simulink subsystem "Final_Project"  (R2024a)
settings: Solver=VariableStepAuto  StartTime=0.0  StopTime=10.0  RelTol=1e-3
undefined symbols (not defined in the file or in its folder): waypoints
libraries: CarMaker4SL x82
(part 3 of 4)

== matlab function Final_Project/Lib_Driving/Subsystem/MATLAB Function1 ==
  data: ego input Bus: EgoStateBus; front_dist output double; lanes input Bus: ParsedLaneBus; traffic input; target_speed input double; ego_lane_id input int32; front_v output double; left_clear output boolean; right_clear output boolean; ego_v input
function [front_dist, front_v, left_clear, right_clear] = traffic_detector(ego, lanes, traffic, target_speed, ego_lane_id, ego_v)
%#codegen
% traffic : Obstacle_Info_Bus
% 내부 구조 예:
%   traffic.t16.x, traffic.t16.y, traffic.t16.vx, traffic.t16.vy
%   ...
%   traffic.t28.x, traffic.t28.y, traffic.t28.vx, traffic.t28.vy
%
% 주의:
%   오류 고친 버전 기준으로 ego_v 입력을 추가함.
%   target_speed는 배선 호환용으로 남겨두지만, 거리 판단에는 ego_v를 사용함.

    unused_target_speed = target_speed; %#ok<NASGU>

    % ============================================================
    % 0. 출력 초기화
    % ============================================================
    front_dist  = 1e9;
    front_v     = 0.0;
    left_clear  = true;
    right_clear = true;
    ego_lane    = int32(ego_lane_id);

    % ============================================================
    % 1. Ego unpack
    % ============================================================
    ego_x = ego.Car_Fr1_tx;
    ego_y = ego.Car_Fr1_ty;

    % ============================================================
    % 2. Lane unpack - 5차선
    % ============================================================
    x1 = lanes.x1; y1 = lanes.y1;
    x2 = lanes.x2; y2 = lanes.y2;
    x3 = lanes.x3; y3 = lanes.y3;
    x4 = lanes.x4; y4 = lanes.y4;
    x5 = lanes.x5; y5 = lanes.y5;

    % detector와 lane5 기준을 맞추기 위한 보정
    L5_OFFSET = 1.0;
    x5 = x5 + L5_OFFSET;

    % ============================================================
    % 3. Ego 속도 기반 가변 탐색/안전거리
    % ============================================================
    v_ego_gap = abs(ego_v);

    % ego_v가 혹시 km/h로 들어오는 경우만 보호
    if v_ego_gap > 60.0
        v_ego_gap = v_ego_gap / 3.6;
    end

    % 같은 차선 앞차 탐색 거리
    LOOK_FRONT = calcLookFront(v_ego_gap);

    % 옆 차선 뒤쪽 안전거리
    CLEAR_BACK_MIN = 5.0;
    CLEAR_BACK_TG  = 0.5;
    CLEAR_BACK_MAX = 35.0;

    CLEAR_BACK = CLEAR_BACK_MIN + CLEAR_BACK_TG * v_ego_gap;

    if CLEAR_BACK > CLEAR_BACK_MAX
        CLEAR_BACK = CLEAR_BACK_MAX;
    end

    % 옆 차선 앞쪽 안전거리
    CLEAR_FRONT_MIN = 15.0;
    CLEAR_FRONT_TG  = 0.9;
    CLEAR_FRONT_MAX = 70.0;

    CLEAR_FRONT = CLEAR_FRONT_MIN + CLEAR_FRONT_TG * v_ego_gap;

    if CLEAR_FRONT > CLEAR_FRONT_MAX
        CLEAR_FRONT = CLEAR_FRONT_MAX;
    end

    % ============================================================
    % 4. Init
    % ============================================================
    front_dist = 1e9;
    front_v    = v_ego_gap;

    left_clear  = true;
    right_clear = true;

    % 도로 끝 차선에서는 없는 방향으로 차선변경 불가 처리
    if ego_lane >= int32(5)
        left_clear = false;
    end

    if ego_lane <= int32(1)
        right_clear = false;
    end

    % ============================================================
    % 5. Traffic_Info_16_Bus ~ Traffic_Info_28_Bus 직접 처리
    % ============================================================
    [front_dist, front_v, left_clear, right_clear] = check_one_signal( ...
        traffic.t16.x, traffic.t16.y, traffic.t16.vx, traffic.t16.vy, true, ...
        ego_x, ego_y, ego_lane, ...
        x1,y1,x2,y2,x3,y3,x4,y4,x5,y5, ...
        front_dist, front_v, left_clear, right_clear, ...
        LOOK_FRONT, CLEAR_BACK, CLEAR_FRONT);

    [front_dist, front_v, left_clear, right_clear] = check_one_signal( ...
        traffic.t17.x, traffic.t17.y, traffic.t17.vx, traffic.t17.vy, true, ...
        ego_x, ego_y, ego_lane, ...
        x1,y1,x2,y2,x3,y3,x4,y4,x5,y5, ...
        front_dist, front_v, left_clear, right_clear, ...
        LOOK_FRONT, CLEAR_BACK, CLEAR_FRONT);

    [front_dist, front_v, left_clear, right_clear] = check_one_signal( ...
        traffic.t18.x, traffic.t18.y, traffic.t18.vx, traffic.t18.vy, true, ...
        ego_x, ego_y, ego_lane, ...
        x1,y1,x2,y2,x3,y3,x4,y4,x5,y5, ...
        front_dist, front_v, left_clear, right_clear, ...
        LOOK_FRONT, CLEAR_BACK, CLEAR_FRONT);

    [front_dist, front_v, left_clear, right_clear] = check_one_signal( ...
        traffic.t19.x, traffic.t19.y, traffic.t19.vx, traffic.t19.vy, true, ...
        ego_x, ego_y, ego_lane, ...
        x1,y1,x2,y2,x3,y3,x4,y4,x5,y5, ...
        front_dist, front_v, left_clear, right_clear, ...
        LOOK_FRONT, CLEAR_BACK, CLEAR_FRONT);

    [front_dist, front_v, left_clear, right_clear] = check_one_signal( ...
        traffic.t20.x, traffic.t20.y, traffic.t20.vx, traffic.t20.vy, true, ...
        ego_x, ego_y, ego_lane, ...
        x1,y1,x2,y2,x3,y3,x4,y4,x5,y5, ...
        front_dist, front_v, left_clear, right_clear, ...
        LOOK_FRONT, CLEAR_BACK, CLEAR_FRONT);

    [front_dist, front_v, left_clear, right_clear] = check_one_signal( ...
        traffic.t21.x, traffic.t21.y, traffic.t21.vx, traffic.t21.vy, true, ...
        ego_x, ego_y, ego_lane, ...
        x1,y1,x2,y2,x3,y3,x4,y4,x5,y5, ...
        front_dist, front_v, left_clear, right_clear, ...
        LOOK_FRONT, CLEAR_BACK, CLEAR_FRONT);

    [front_dist, front_v, left_clear, right_clear] = check_one_signal( ...
        traffic.t22.x, traffic.t22.y, traffic.t22.vx, traffic.t22.vy, true, ...
        ego_x, ego_y, ego_lane, ...
        x1,y1,x2,y2,x3,y3,x4,y4,x5,y5, ...
        front_dist, front_v, left_clear, right_clear, ...
        LOOK_FRONT, CLEAR_BACK, CLEAR_FRONT);

    [front_dist, front_v, left_clear, right_clear] = check_one_signal( ...
        traffic.t23.x, traffic.t23.y, traffic.t23.vx, traffic.t23.vy, true, ...
        ego_x, ego_y, ego_lane, ...
        x1,y1,x2,y2,x3,y3,x4,y4,x5,y5, ...
        front_dist, front_v, left_clear, right_clear, ...
        LOOK_FRONT, CLEAR_BACK, CLEAR_FRONT);

    [front_dist, front_v, left_clear, right_clear] = check_one_signal( ...
        traffic.t24.x, traffic.t24.y, traffic.t24.vx, traffic.t24.vy, true, ...
        ego_x, ego_y, ego_lane, ...
        x1,y1,x2,y2,x3,y3,x4,y4,x5,y5, ...
        front_dist, front_v, left_clear, right_clear, ...
        LOOK_FRONT, CLEAR_BACK, CLEAR_FRONT);

    [front_dist, front_v, left_clear, right_clear] = check_one_signal( ...
        traffic.t25.x, traffic.t25.y, traffic.t25.vx, traffic.t25.vy, true, ...
        ego_x, ego_y, ego_lane, ...
        x1,y1,x2,y2,x3,y3,x4,y4,x5,y5, ...
        front_dist, front_v, left_clear, right_clear, ...
        LOOK_FRONT, CLEAR_BACK, CLEAR_FRONT);

    [front_dist, front_v, left_clear, right_clear] = check_one_signal( ...
        traffic.t26.x, traffic.t26.y, traffic.t26.vx, traffic.t26.vy, true, ...
        ego_x, ego_y, ego_lane, ...
        x1,y1,x2,y2,x3,y3,x4,y4,x5,y5, ...
        front_dist, front_v, left_clear, right_clear, ...
        LOOK_FRONT, CLEAR_BACK, CLEAR_FRONT);

    [front_dist, front_v, left_clear, right_clear] = check_one_signal( ...
        traffic.t27.x, traffic.t27.y, traffic.t27.vx, traffic.t27.vy, true, ...
        ego_x, ego_y, ego_lane, ...
        x1,y1,x2,y2,x3,y3,x4,y4,x5,y5, ...
        front_dist, front_v, left_clear, right_clear, ...
        LOOK_FRONT, CLEAR_BACK, CLEAR_FRONT);

    [front_dist, front_v, left_clear, right_clear] = check_one_signal( ...
        traffic.t28.x, traffic.t28.y, traffic.t28.vx, traffic.t28.vy, true, ...
        ego_x, ego_y, ego_lane, ...
        x1,y1,x2,y2,x3,y3,x4,y4,x5,y5, ...
        front_dist, front_v, left_clear, right_clear, ...
        LOOK_FRONT, CLEAR_BACK, CLEAR_FRONT);

end


function LOOK_FRONT = calcLookFront(v)
%#codegen
    v = abs(v);

    if v > 60.0
        v = v / 3.6;
    end

    % 80 km/h 기준으로 고속 구간 탐색거리 급격히 확대
    V_HIGH = 80.0 / 3.6;

    if v < V_HIGH
        LOOK_FRONT = 25.0 + 1.0 * v;
    else
        LOOK_FRONT = 25.0 + 1.0 * V_HIGH + 10.0 * (v - V_HIGH);
    end

    if LOOK_FRONT > 120.0
        LOOK_FRONT = 120.0;
    end
end


function [front_dist, front_v, left_clear, right_clear] = check_one_signal( ...
    obj_x, obj_y, obj_vx, obj_vy, valid, ...
    ego_x, ego_y, ego_lane_id, ...
    x1,y1,x2,y2,x3,y3,x4,y4,x5,y5, ...
    front_dist, front_v, left_clear, right_clear, ...
    LOOK_FRONT, CLEAR_BACK, CLEAR_FRONT)
%#codegen

    if ~valid
        return;
    end

    [front_dist, front_v, left_clear, right_clear] = check_one_vehicle( ...
        ego_x, ego_y, ego_lane_id, ...
        obj_x, obj_y, obj_vx, obj_vy, ...
        x1,y1,x2,y2,x3,y3,x4,y4,x5,y5, ...
        front_dist, front_v, left_clear, right_clear, ...
        LOOK_FRONT, CLEAR_BACK, CLEAR_FRONT);

end


function [front_dist, front_v, left_clear, right_clear] = check_one_vehicle( ...
    ego_x, ego_y, ego_lane_id, ...
    obj_x, obj_y, obj_vx, obj_vy, ...
    x1, y1, x2, y2, x3, y3, x4, y4, x5, y5, ...
    front_dist, front_v, left_clear, right_clear, ...
    LOOK_FRONT, CLEAR_BACK, CLEAR_FRONT)
%#codegen

    % Object가 어느 차선에 가장 가까운지 판단
    [obj_lane_id, obj_idx] = nearest_lane_id( ...
        obj_x, obj_y, ...
        x1, y1, x2, y2, x3, y3, x4, y4, x5, y5);

    % ============================================================
    % 1. 같은 차선 앞차 판단
    % lane 1,2,3은 순환트랙 forward 거리 사용
    % lane 4,5는 비순환 signed 거리 사용
    % ============================================================
    if obj_lane_id == ego_lane_id

        ego_idx = nearest_idx_by_lane( ...
            ego_lane_id, ego_x, ego_y, ...
            x1, y1, x2, y2, x3, y3, x4, y4, x5, y5);

        s_rel = arc_dist_forward_by_lane( ...
            ego_lane_id, ego_idx, obj_idx, ...
            x1, y1, x2, y2, x3, y3, x4, y4, x5, y5);

        if s_rel > 0.0 && s_rel < LOOK_FRONT
            if s_rel < front_dist
                front_dist = s_rel;
                front_v = sqrt(obj_vx*obj_vx + obj_vy*obj_vy);
            end
        end
    end

    % ============================================================
    % 2. 왼쪽 인접 차선 차량 확인
    % 차선 번호 증가 방향 = 왼쪽
    % ============================================================
    if obj_lane_id == ego_lane_id + int32(1)

        ego_idx_adj = nearest_idx_by_lane( ...
            obj_lane_id, ego_x, ego_y, ...
            x1, y1, x2, y2, x3, y3, x4, y4, x5, y5);

        is_close = is_close_on_adj_lane( ...
            obj_lane_id, ego_idx_adj, obj_idx, ...
            CLEAR_BACK, CLEAR_FRONT, ...
            x1, y1, x2, y2, x3, y3, x4, y4, x5, y5);

        if is_close
            left_clear = false;
        end

    % ============================================================
    % 3. 오른쪽 인접 차선 차량 확인
    % 차선 번호 감소 방향 = 오른쪽
    % ============================================================
    elseif obj_lane_id == ego_lane_id - int32(1)

        ego_idx_adj = nearest_idx_by_lane( ...
            obj_lane_id, ego_x, ego_y, ...
            x1, y1, x2, y2, x3, y3, x4, y4, x5, y5);

        is_close = is_close_on_adj_lane( ...
            obj_lane_id, ego_idx_adj, obj_idx, ...
            CLEAR_BACK, CLEAR_FRONT, ...
            x1, y1, x2, y2, x3, y3, x4, y4, x5, y5);

        if is_close
            right_clear = false;
        end
    end

end


function [lane_id, best_idx] = nearest_lane_id(px, py, x1, y1, x2, y2, x3, y3, x4, y4, x5, y5)
%#codegen

    [idx1, d1] = nearest_idx_d2(x1, y1, px, py);
    [idx2, d2] = nearest_idx_d2(x2, y2, px, py);
    [idx3, d3] = nearest_idx_d2(x3, y3, px, py);
    [idx4, d4] = nearest_idx_d2(x4, y4, px, py);
    [idx5, d5] = nearest_idx_d2(x5, y5, px, py);

    lane_id  = int32(1);
    best_idx = idx1;
    best_d2  = d1;

    if d2 < best_d2
        lane_id  = int32(2);
        best_idx = idx2;
        best_d2  = d2;
    end

    if d3 < best_d2
        lane_id  = int32(3);
        best_idx = idx3;
        best_d2  = d3;
    end

    if d4 < best_d2
        lane_id  = int32(4);
        best_idx = idx4;
        best_d2  = d4;
    end

    if d5 < best_d2
        lane_id  = int32(5);
        best_idx = idx5;
    end

end


function idx = nearest_idx_by_lane(lane_id, px, py, x1, y1, x2, y2, x3, y3, x4, y4, x5, y5)
%#codegen

    if lane_id == int32(1)
        [idx, ~] = nearest_idx_d2(x1, y1, px, py);
    elseif lane_id == int32(2)
        [idx, ~] = nearest_idx_d2(x2, y2, px, py);
    elseif lane_id == int32(3)
        [idx, ~] = nearest_idx_d2(x3, y3, px, py);
    elseif lane_id == int32(4)
        [idx, ~] = nearest_idx_d2(x4, y4, px, py);
    else
        [idx, ~] = nearest_idx_d2(x5, y5, px, py);
    end

end


function [best_i, best_d2] = nearest_idx_d2(xa, ya, px, py)
%#codegen

    best_i  = int32(1);
    best_d2 = 1e12;
    N = int32(numel(xa));

    for i = 1:N
        dx = xa(i) - px;
        dy = ya(i) - py;
        d2 = dx*dx + dy*dy;

        if d2 < best_d2
            best_d2 = d2;
            best_i  = i;
        end
    end

end


function ds = arc_dist_forward_by_lane(lane_id, idx_from, idx_to, ...
    x1, y1, x2, y2, x3, y3, x4, y4, x5, y5)
%#codegen
% 앞차 판단 전용 forward distance
% lane 1,2,3은 순환트랙으로 보고 wrap-around 거리 계산
% lane 4,5는 비순환 차선으로 보고 기존 signed arc distance 사용

    if lane_id == int32(1)
        ds = arc_dist_forward_closed(x1, y1, idx_from, idx_to);
    elseif lane_id == int32(2)
        ds = arc_dist_forward_closed(x2, y2, idx_from, idx_to);
    elseif lane_id == int32(3)
        ds = arc_dist_forward_closed(x3, y3, idx_from, idx_to);
    elseif lane_id == int32(4)
        ds = arc_dist_open(x4, y4, idx_from, idx_to);
    else
        ds = arc_dist_open(x5, y5, idx_from, idx_to);
    end

end


function ds = arc_dist_forward_closed(xa, ya, idx_from, idx_to)
%#codegen
% 순환트랙용 전방 arc distance
% idx_to < idx_from이어도 끝점 -> 시작점으로 이어서 양수 거리 계산

    ds = 0.0;
    N = int32(numel(xa));

    if idx_to == idx_from
        ds = 0.0;
        return;
    end

    if idx_to > idx_from

        for i = idx_from:(idx_to - int32(1))
            dx = xa(i+1) - xa(i);
            dy = ya(i+1) - ya(i);
            ds = ds + sqrt(dx*dx + dy*dy);
        end

    else

        for i = idx_from:(N - int32(1))
            dx = xa(i+1) - xa(i);
            dy = ya(i+1) - ya(i);
            ds = ds + sqrt(dx*dx + dy*dy);
        end

        % 마지막 waypoint -> 첫 번째 waypoint 연결
        dx = xa(1) - xa(N);
        dy = ya(1) - ya(N);
        ds = ds + sqrt(dx*dx + dy*dy);

        for i = int32(1):(idx_to - int32(1))
            dx = xa(i+1) - xa(i);
            dy = ya(i+1) - ya(i);
            ds = ds + sqrt(dx*dx + dy*dy);
        end

    end

end


function is_close = is_close_on_adj_lane(lane_id, idx_from, idx_to, ...
    CLEAR_BACK, CLEAR_FRONT, ...
    x1, y1, x2, y2, x3, y3, x4, y4, x5, y5)
%#codegen
% 옆차선 clear 판단용 거리 계산
%
% lane 1,2,3:
%   순환트랙으로 보고 forward/backward 거리 둘 다 확인
%
% lane 4,5:
%   비순환 차선으로 보고 signed 거리 사용

    is_close = false;

    if lane_id == int32(1)

        fwd_dist  = arc_dist_forward_closed(x1, y1, idx_from, idx_to);
        total_len = arc_length_closed(x1, y1);
        back_dist = total_len - fwd_dist;

        if fwd_dist < CLEAR_FRONT || back_dist < CLEAR_BACK
            is_close = true;
        end

    elseif lane_id == int32(2)

        fwd_dist  = arc_dist_forward_closed(x2, y2, idx_from, idx_to);
        total_len = arc_length_closed(x2, y2);
        back_dist = total_len - fwd_dist;

        if fwd_dist < CLEAR_FRONT || back_dist < CLEAR_BACK
            is_close = true;
        end

    elseif lane_id == int32(3)

        fwd_dist  = arc_dist_forward_closed(x3, y3, idx_from, idx_to);
        total_len = arc_length_closed(x3, y3);
        back_dist = total_len - fwd_dist;

        if fwd_dist < CLEAR_FRONT || back_dist < CLEAR_BACK
            is_close = true;
        end

    elseif lane_id == int32(4)

        s_rel = arc_dist_open(x4, y4, idx_from, idx_to);

        if s_rel > -CLEAR_BACK && s_rel < CLEAR_FRONT
            is_close = true;
        end

    else

        s_rel = arc_dist_open(x5, y5, idx_from, idx_to);

        if s_rel > -CLEAR_BACK && s_rel < CLEAR_FRONT
            is_close = true;
        end

    end

end


function total_len = arc_length_closed(xa, ya)
%#codegen
% 순환트랙 전체 길이 계산
% 마지막 waypoint -> 첫 번째 waypoint 연결까지 포함

    total_len = 0.0;
    N = int32(numel(xa));

    for i = int32(1):(N - int32(1))
        dx = xa(i+1) - xa(i);
        dy = ya(i+1) - ya(i);
        total_len = total_len + sqrt(dx*dx + dy*dy);
    end

    dx = xa(1) - xa(N);
    dy = ya(1) - ya(N);
    total_len = total_len + sqrt(dx*dx + dy*dy);

end


function ds = arc_dist_open(xa, ya, idx_from, idx_to)
%#codegen
% 비순환 signed arc distance
% idx_to > idx_from : 양수
% idx_to < idx_from : 음수

    ds = 0.0;

    if idx_to == idx_from

        ds = 0.0;

    elseif idx_to > idx_from

        for i = idx_from:(idx_to - int32(1))
            dx = xa(i+1) - xa(i);
            dy = ya(i+1) - ya(i);
            ds = ds + sqrt(dx*dx + dy*dy);
        end

    else

        for i = idx_to:(idx_from - int32(1))
            dx = xa(i+1) - xa(i);
            dy = ya(i+1) - ya(i);
            ds = ds - sqrt(dx*dx + dy*dy);
        end

    end

end

% function [front_dist, front_v, left_clear, right_clear] = traffic_detector(ego, lanes, traffic, target_speed, ego_lane_id)
% %#codegen
% % traffic : Obstacle_Info_Bus
% % 내부 구조:
% %   traffic.t16.x
% %   traffic.t16.y
% %   traffic.t16.vx
% %   traffic.t16.vy
% %   ...
% %   traffic.t28.x
% %   traffic.t28.y
% %   traffic.t28.vx
% %   traffic.t28.vy
% 
%     % ============================================================
%     % 0. 출력 초기화
%     % Simulink가 출력 타입을 확정할 수 있게 명시
%     % ============================================================
%     front_dist  = 1e9;
%     front_v     = 0.0;
%     left_clear  = true;
%     right_clear = true;
%     ego_lane    = int32(ego_lane_id);
% 
%     % ============================================================
%     % 1. Ego unpack
%     % ============================================================
%     ego_x = ego.Car_Fr1_tx;
%     ego_y = ego.Car_Fr1_ty;
% 
%     % ============================================================
%     % 2. Lane unpack - 5차선
%     % ============================================================
%     x1 = lanes.x1; y1 = lanes.y1;
%     x2 = lanes.x2; y2 = lanes.y2;
%     x3 = lanes.x3; y3 = lanes.y3;
%     x4 = lanes.x4; y4 = lanes.y4;
%     x5 = lanes.x5; y5 = lanes.y5;
% 
%     % ============================================================
%     % 3. Parameters - Ego 속도 기반 가변 탐색/안전거리
%     %
%     % 현재 함수 입력에는 ego_v가 따로 없으므로 target_speed를
%     % ego 기준 속도로 사용함.
%     %
%     % target_speed가 km/h로 들어오면 m/s로 변환한다.
%     % 판단 기준:
%     %   20보다 크면 km/h로 보고 /3.6
%     %   20 이하면 m/s로 사용
%     % ============================================================
%     v_ego_gap = abs(target_speed);
% 
%     if v_ego_gap > 20.0
%         v_ego_gap = v_ego_gap / 3.6;
%     end
% 
%     % -----------------------------
%     % 1) 같은 차선 앞차 탐색 거리
%     % 거리 = 최소거리 + 속도 * 타임갭
%     % -----------------------------
%     LOOK_FRONT_MIN = 20.0;   % 최소 앞차 탐색거리 [m]
%     LOOK_FRONT_TG  = 1.5;    % 앞차 탐색 time gap [s]
%     LOOK_FRONT_MAX = 80.0;   % 최대 앞차 탐색거리 [m]
% 
%     LOOK_FRONT = LOOK_FRONT_MIN + LOOK_FRONT_TG * v_ego_gap;
% 
%     if LOOK_FRONT > LOOK_FRONT_MAX
%         LOOK_FRONT = LOOK_FRONT_MAX;
%     end
% 
%     % -----------------------------
%     % 2) 옆 차선 뒤쪽 안전거리
%     % -----------------------------
%     CLEAR_BACK_MIN = 5.0;    % 최소 후방 안전거리 [m]
%     CLEAR_BACK_TG  = 0.7;    % 후방 time gap [s]
%     CLEAR_BACK_MAX = 35.0;   % 최대 후방 안전거리 [m]
% 
%     CLEAR_BACK = CLEAR_BACK_MIN + CLEAR_BACK_TG * v_ego_gap;
% 
%     if CLEAR_BACK > CLEAR_BACK_MAX
%         CLEAR_BACK = CLEAR_BACK_MAX;
%     end
% 
%     % -----------------------------
%     % 3) 옆 차선 앞쪽 안전거리
%     % -----------------------------
%     CLEAR_FRONT_MIN = 15.0;  % 최소 전방 안전거리 [m]
%     CLEAR_FRONT_TG  = 1.2;   % 전방 time gap [s]
%     CLEAR_FRONT_MAX = 70.0;  % 최대 전방 안전거리 [m]
% 
%     CLEAR_FRONT = CLEAR_FRONT_MIN + CLEAR_FRONT_TG * v_ego_gap;
% 
%     if CLEAR_FRONT > CLEAR_FRONT_MAX
%         CLEAR_FRONT = CLEAR_FRONT_MAX;
%     end
% 
%     % ============================================================
%     % 4. Init
%     % ============================================================
%     front_dist = 1e9;
% 
%     % 앞차가 없을 때의 기본 front_v
%     % 위에서 단위 변환된 ego 기준 속도를 사용
%     front_v = v_ego_gap;
% 
%     left_clear  = true;
%     right_clear = true;
% 
%     % 도로 끝 차선에서는 없는 방향으로 차선변경 불가 처리
%     if ego_lane >= int32(5)
%         left_clear = false;
%     end
% 
%     if ego_lane <= int32(1)
%         right_clear = false;
%     end
% 
%     % ============================================================
%     % 5. Traffic_Info_16_Bus ~ Traffic_Info_28_Bus 직접 처리
%     % ============================================================
% 
%     [front_dist, front_v, left_clear, right_clear] = check_one_signal( ...
%         traffic.t16.x, traffic.t16.y, ...
%         traffic.t16.vx, traffic.t16.vy, true, ...
%         ego_x, ego_y, ego_lane, ...
%         x1,y1,x2,y2,x3,y3,x4,y4,x5,y5, ...
%         front_dist, front_v, left_clear, right_clear, ...
%         LOOK_FRONT, CLEAR_BACK, CLEAR_FRONT);
% 
%     [front_dist, front_v, left_clear, right_clear] = check_one_signal( ...
%         traffic.t17.x, traffic.t17.y, ...
%         traffic.t17.vx, traffic.t17.vy, true, ...
%         ego_x, ego_y, ego_lane, ...
%         x1,y1,x2,y2,x3,y3,x4,y4,x5,y5, ...
%         front_dist, front_v, left_clear, right_clear, ...
%         LOOK_FRONT, CLEAR_BACK, CLEAR_FRONT);
% 
%     [front_dist, front_v, left_clear, right_clear] = check_one_signal( ...
%         traffic.t18.x, traffic.t18.y, ...
%         traffic.t18.vx, traffic.t18.vy, true, ...
%         ego_x, ego_y, ego_lane, ...
%         x1,y1,x2,y2,x3,y3,x4,y4,x5,y5, ...
%         front_dist, front_v, left_clear, right_clear, ...
%         LOOK_FRONT, CLEAR_BACK, CLEAR_FRONT);
% 
%     [front_dist, front_v, left_clear, right_clear] = check_one_signal( ...
%         traffic.t19.x, traffic.t19.y, ...
%         traffic.t19.vx, traffic.t19.vy, true, ...
%         ego_x, ego_y, ego_lane, ...
%         x1,y1,x2,y2,x3,y3,x4,y4,x5,y5, ...
%         front_dist, front_v, left_clear, right_clear, ...
%         LOOK_FRONT, CLEAR_BACK, CLEAR_FRONT);
% 
%     [front_dist, front_v, left_clear, right_clear] = check_one_signal( ...
%         traffic.t20.x, traffic.t20.y, ...
%         traffic.t20.vx, traffic.t20.vy, true, ...
%         ego_x, ego_y, ego_lane, ...
%         x1,y1,x2,y2,x3,y3,x4,y4,x5,y5, ...
%         front_dist, front_v, left_clear, right_clear, ...
%         LOOK_FRONT, CLEAR_BACK, CLEAR_FRONT);
% 
%     [front_dist, front_v, left_clear, right_clear] = check_one_signal( ...
%         traffic.t21.x, traffic.t21.y, ...
%         traffic.t21.vx, traffic.t21.vy, true, ...
%         ego_x, ego_y, ego_lane, ...
%         x1,y1,x2,y2,x3,y3,x4,y4,x5,y5, ...
%         front_dist, front_v, left_clear, right_clear, ...
%         LOOK_FRONT, CLEAR_BACK, CLEAR_FRONT);
% 
%     [front_dist, front_v, left_clear, right_clear] = check_one_signal( ...
%         traffic.t22.x, traffic.t22.y, ...
%         traffic.t22.vx, traffic.t22.vy, true, ...
%         ego_x, ego_y, ego_lane, ...
%         x1,y1,x2,y2,x3,y3,x4,y4,x5,y5, ...
%         front_dist, front_v, left_clear, right_clear, ...
%         LOOK_FRONT, CLEAR_BACK, CLEAR_FRONT);
% 
%     [front_dist, front_v, left_clear, right_clear] = check_one_signal( ...
%         traffic.t23.x, traffic.t23.y, ...
%         traffic.t23.vx, traffic.t23.vy, true, ...
%         ego_x, ego_y, ego_lane, ...
%         x1,y1,x2,y2,x3,y3,x4,y4,x5,y5, ...
%         front_dist, front_v, left_clear, right_clear, ...
%         LOOK_FRONT, CLEAR_BACK, CLEAR_FRONT);
% 
%     [front_dist, front_v, left_clear, right_clear] = check_one_signal( ...
%         traffic.t24.x, traffic.t24.y, ...
%         traffic.t24.vx, traffic.t24.vy, true, ...
%         ego_x, ego_y, ego_lane, ...
%         x1,y1,x2,y2,x3,y3,x4,y4,x5,y5, ...
%         front_dist, front_v, left_clear, right_clear, ...
%         LOOK_FRONT, CLEAR_BACK, CLEAR_FRONT);
% 
%     [front_dist, front_v, left_clear, right_clear] = check_one_signal( ...
%         traffic.t25.x, traffic.t25.y, ...
%         traffic.t25.vx, traffic.t25.vy, true, ...
%         ego_x, ego_y, ego_lane, ...
%         x1,y1,x2,y2,x3,y3,x4,y4,x5,y5, ...
%         front_dist, front_v, left_clear, right_clear, ...
%         LOOK_FRONT, CLEAR_BACK, CLEAR_FRONT);
% 
%     [front_dist, front_v, left_clear, right_clear] = check_one_signal( ...
%         traffic.t26.x, traffic.t26.y, ...
%         traffic.t26.vx, traffic.t26.vy, true, ...
%         ego_x, ego_y, ego_lane, ...
%         x1,y1,x2,y2,x3,y3,x4,y4,x5,y5, ...
%         front_dist, front_v, left_clear, right_clear, ...
%         LOOK_FRONT, CLEAR_BACK, CLEAR_FRONT);
% 
%     [front_dist, front_v, left_clear, right_clear] = check_one_signal( ...
%         traffic.t27.x, traffic.t27.y, ...
%         traffic.t27.vx, traffic.t27.vy, true, ...
%         ego_x, ego_y, ego_lane, ...
%         x1,y1,x2,y2,x3,y3,x4,y4,x5,y5, ...
%         front_dist, front_v, left_clear, right_clear, ...
%         LOOK_FRONT, CLEAR_BACK, CLEAR_FRONT);
% 
%     [front_dist, front_v, left_clear, right_clear] = check_one_signal( ...
%         traffic.t28.x, traffic.t28.y, ...
%         traffic.t28.vx, traffic.t28.vy, true, ...
%         ego_x, ego_y, ego_lane, ...
%         x1,y1,x2,y2,x3,y3,x4,y4,x5,y5, ...
%         front_dist, front_v, left_clear, right_clear, ...
%         LOOK_FRONT, CLEAR_BACK, CLEAR_FRONT);
% 
% end
% 
% 
% function [front_dist, front_v, left_clear, right_clear] = check_one_signal( ...
%     obj_x, obj_y, obj_vx, obj_vy, valid, ...
%     ego_x, ego_y, ego_lane_id, ...
%     x1,y1,x2,y2,x3,y3,x4,y4,x5,y5, ...
%     front_dist, front_v, left_clear, right_clear, ...
%     LOOK_FRONT, CLEAR_BACK, CLEAR_FRONT)
% %#codegen
% 
%     if ~valid
%         return;
%     end
% 
%     [front_dist, front_v, left_clear, right_clear] = check_one_vehicle( ...
%         ego_x, ego_y, ego_lane_id, ...
%         obj_x, obj_y, obj_vx, obj_vy, ...
%         x1,y1,x2,y2,x3,y3,x4,y4,x5,y5, ...
%         front_dist, front_v, left_clear, right_clear, ...
%         LOOK_FRONT, CLEAR_BACK, CLEAR_FRONT);
% 
% end
% 
% 
% function [front_dist, front_v, left_clear, right_clear] = check_one_vehicle( ...
%     ego_x, ego_y, ego_lane_id, ...
%     obj_x, obj_y, obj_vx, obj_vy, ...
%     x1, y1, x2, y2, x3, y3, x4, y4, x5, y5, ...
%     front_dist, front_v, left_clear, right_clear, ...
%     LOOK_FRONT, CLEAR_BACK, CLEAR_FRONT)
% %#codegen
% 
%     % ============================================================
%     % Object가 어느 차선에 가장 가까운지 판단
%     % ============================================================
%     [obj_lane_id, obj_idx] = nearest_lane_id( ...
%         obj_x, obj_y, ...
%         x1, y1, x2, y2, x3, y3, x4, y4, x5, y5);
% 
%     % ============================================================
%     % 1. 같은 차선 차량이면 front vehicle 후보
%     % ============================================================
%     if obj_lane_id == ego_lane_id
% 
%         ego_idx = nearest_idx_by_lane( ...
%             ego_lane_id, ego_x, ego_y, ...
%             x1, y1, x2, y2, x3, y3, x4, y4, x5, y5);
% 
%         s_rel = arc_dist_by_lane( ...
%             ego_lane_id, ego_idx, obj_idx, ...
%             x1, y1, x2, y2, x3, y3, x4, y4, x5, y5);
% 
%         if s_rel > 0.0 && s_rel < LOOK_FRONT
%             if s_rel < front_dist
%                 front_dist = s_rel;
%                 front_v = sqrt(obj_vx*obj_vx + obj_vy*obj_vy);
%             end
%         end
% 
%     % ============================================================
%     % 2. 왼쪽 인접 차선 차량 확인
%     % lane 번호가 커지는 방향을 왼쪽으로 가정
%     % ============================================================
%     elseif obj_lane_id == ego_lane_id + int32(1)
% 
%         ego_idx_adj = nearest_idx_by_lane( ...
%             obj_lane_id, ego_x, ego_y, ...
%             x1, y1, x2, y2, x3, y3, x4, y4, x5, y5);
% 
%         s_rel = arc_dist_by_lane( ...
%             obj_lane_id, ego_idx_adj, obj_idx, ...
%             x1, y1, x2, y2, x3, y3, x4, y4, x5, y5);
% 
%         if s_rel > -CLEAR_BACK && s_rel < CLEAR_FRONT
%             left_clear = false;
%         end
% 
%     % ============================================================
%     % 3. 오른쪽 인접 차선 차량 확인
%     % lane 번호가 작아지는 방향을 오른쪽으로 가정
%     % ============================================================
%     elseif obj_lane_id == ego_lane_id - int32(1)
% 
%         ego_idx_adj = nearest_idx_by_lane( ...
%             obj_lane_id, ego_x, ego_y, ...
%             x1, y1, x2, y2, x3, y3, x4, y4, x5, y5);
% 
%         s_rel = arc_dist_by_lane( ...
%             obj_lane_id, ego_idx_adj, obj_idx, ...
%             x1, y1, x2, y2, x3, y3, x4, y4, x5, y5);
% 
%         if s_rel > -CLEAR_BACK && s_rel < CLEAR_FRONT
%             right_clear = false;
%         end
%     end
% 
% end
% 
% 
% function [lane_id, best_idx] = nearest_lane_id(px, py, x1, y1, x2, y2, x3, y3, x4, y4, x5, y5)
% %#codegen
% 
%     [idx1, d1] = nearest_idx_d2(x1, y1, px, py);
%     [idx2, d2] = nearest_idx_d2(x2, y2, px, py);
%     [idx3, d3] = nearest_idx_d2(x3, y3, px, py);
%     [idx4, d4] = nearest_idx_d2(x4, y4, px, py);
%     [idx5, d5] = nearest_idx_d2(x5, y5, px, py);
% 
%     lane_id  = int32(1);
%     best_idx = idx1;
%     best_d2  = d1;
% 
%     if d2 < best_d2
%         lane_id  = int32(2);
%         best_idx = idx2;
%         best_d2  = d2;
%     end
% 
%     if d3 < best_d2
%         lane_id  = int32(3);
%         best_idx = idx3;
%         best_d2  = d3;
%     end
% 
%     if d4 < best_d2
%         lane_id  = int32(4);
%         best_idx = idx4;
%         best_d2  = d4;
%     end
% 
%     if d5 < best_d2
%         lane_id  = int32(5);
%         best_idx = idx5;
%     end
% 
% end
% 
% 
% function idx = nearest_idx_by_lane(lane_id, px, py, x1, y1, x2, y2, x3, y3, x4, y4, x5, y5)
% %#codegen
% 
%     if lane_id == int32(1)
%         [idx, ~] = nearest_idx_d2(x1, y1, px, py);
%     elseif lane_id == int32(2)
%         [idx, ~] = nearest_idx_d2(x2, y2, px, py);
%     elseif lane_id == int32(3)
%         [idx, ~] = nearest_idx_d2(x3, y3, px, py);
%     elseif lane_id == int32(4)
%         [idx, ~] = nearest_idx_d2(x4, y4, px, py);
%     else
%         [idx, ~] = nearest_idx_d2(x5, y5, px, py);
%     end
% 
% end
% 
% 
% function [best_i, best_d2] = nearest_idx_d2(xa, ya, px, py)
% %#codegen
% 
%     best_i  = int32(1);
%     best_d2 = 1e12;
% 
%     N = int32(numel(xa));
% 
%     for i = 1:N
%         dx = xa(i) - px;
%         dy = ya(i) - py;
%         d2 = dx*dx + dy*dy;
% 
%         if d2 < best_d2
%             best_d2 = d2;
%             best_i  = i;
%         end
%     end
% 
% end
% 
% 
% function ds = arc_dist_by_lane(lane_id, idx_from, idx_to, x1, y1, x2, y2, x3, y3, x4, y4, x5, y5)
% %#codegen
% 
%     if lane_id == int32(1)
%         ds = arc_dist(x1, y1, idx_from, idx_to);
%     elseif lane_id == int32(2)
%         ds = arc_dist(x2, y2, idx_from, idx_to);
%     elseif lane_id == int32(3)
%         ds = arc_dist(x3, y3, idx_from, idx_to);
%     elseif lane_id == int32(4)
%         ds = arc_dist(x4, y4, idx_from, idx_to);
%     else
%         ds = arc_dist(x5, y5, idx_from, idx_to);
%     end
% 
% end
% 
% 
% function ds = arc_dist(xa, ya, idx_from, idx_to)
% %#codegen
% 
%     ds = 0.0;
% 
%     if idx_to == idx_from
% 
%         ds = 0.0;
% 
%     elseif idx_to > idx_from
% 
%         for i = idx_from:(idx_to - int32(1))
%             dx = xa(i+1) - xa(i);
%             dy = ya(i+1) - ya(i);
%             ds = ds + sqrt(dx*dx + dy*dy);
%         end
% 
%     else
% 
%         for i = idx_to:(idx_from - int32(1))
%             dx = xa(i+1) - xa(i);
%             dy = ya(i+1) - ya(i);
%             ds = ds - sqrt(dx*dx + dy*dy);
%         end
% 
%     end
% 
% end
